simulink model "Android_interface_2Aero"  (R2018b)
settings: Solver=FixedStepDiscrete  StartTime=0.0  StopTime=inf  FixedStep=0.002  RelTol=1e-3
libraries: androiduilib x8, androidcommunicationlib x8
settings Model: SimulationMode=external  ExtModeTrigDuration=10000  Creator=gjaniak  LastModifiedBy=gjaniak
settings SolverCC: PositivePriorityOrder=on
settings OptimizationCC: PassReuseOutputArgsThreshold=0  MaxStackSize=64
settings DebuggingCC: ParameterTunabilityLossMsg=error  LibraryContextMissingDiagnostic=none
settings HardwareCC: ProdBitPerPointer=32  ProdBitPerSizeT=32  ProdBitPerPtrDiffT=32  ProdLargestAtomicInteger=Long  ProdLargestAtomicFloat=Double  ProdWordSize=32  ProdHWDeviceType=ARM Compatible->ARM Cortex  UseEmbeddedCoderFeatures=off
settings SFSimCC: SimUseLocalCustomCode=off
settings RTWCC: SystemTargetFile=ert.tlc  HardwareBoard=Android Device  TLCOptions="-aInlineSetEventsForThisBaseRateFcn=TLC_FALSE -aSuppressMultiTaskScheduler=TLC_FALSE  -aRateBasedStepFcn=0"  TemplateMakefile=ert_default_tmf  GenerateReport=on  RTWUseLocalCustomCode=off  Toolchain=Android SDK/NDK Tools  LaunchReport=on
settings CodeAppCC: ForceParamTrailComments=on  OperatorAnnotations=on  StateflowObjectComments=on  MATLABSourceComments=on
settings ERTTargetCC: MultiwordLength=2048  ERTCustomFileBanners=off  SupportContinuousTime=on  SupportNonInlinedSFcns=on  RemoveResetFunc=off  ModelStepFunctionPrototypeControlCompliant=off

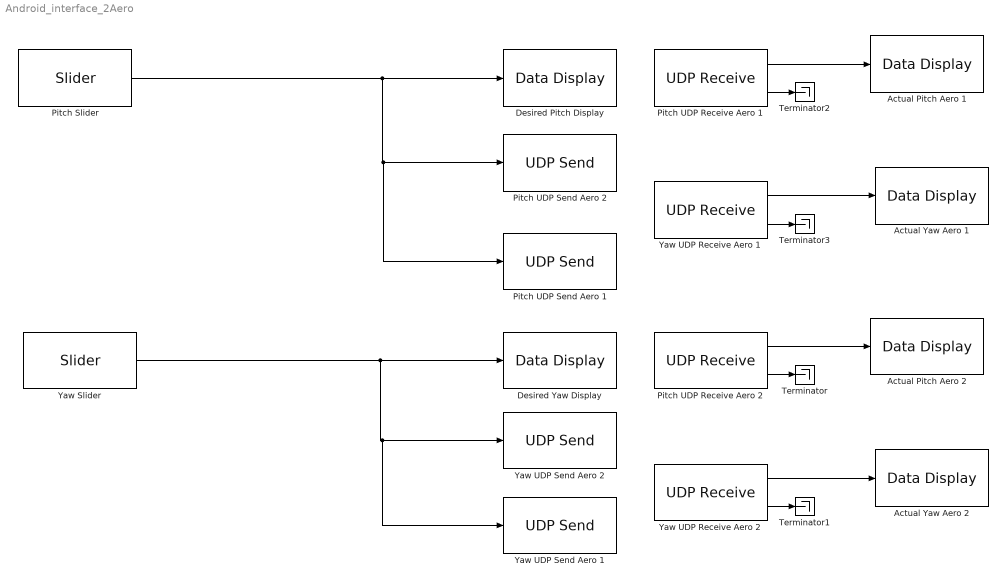
== system Android_interface_2Aero ==
  Actual Pitch Aero 1 : androiduilib/Data Display  DataDisplayId=Android_interface_2Aero/Actual_Pitch_Aero_1  Format=Float  Precision=6  SimulateUsing=Code generation  blockPlatform=Android
      settings: SourceProductName=Simulink Support Package for Android Devices  SourceProductBaseCode=ANDROID
  Actual Pitch Aero 2 : androiduilib/Data Display  DataDisplayId=Android_interface_2Aero/Actual_Pitch_Aero_2  Format=Float  Precision=6  SimulateUsing=Code generation  blockPlatform=Android
      settings: SourceProductName=Simulink Support Package for Android Devices  SourceProductBaseCode=ANDROID
  Actual Yaw Aero 1 : androiduilib/Data Display  DataDisplayId=Android_interface_2Aero/Actual_Yaw_Aero_1  Format=Float  Precision=6  SimulateUsing=Code generation  blockPlatform=Android
      settings: SourceProductName=Simulink Support Package for Android Devices  SourceProductBaseCode=ANDROID
  Actual Yaw Aero 2 : androiduilib/Data Display  DataDisplayId=Android_interface_2Aero/Actual_Yaw_Aero_2  Format=Float  Precision=6  SimulateUsing=Code generation  blockPlatform=Android
      settings: SourceProductName=Simulink Support Package for Android Devices  SourceProductBaseCode=ANDROID
  Desired Pitch Display : androiduilib/Data Display  DataDisplayId=Android_interface_2Aero/Desired_Pitch_Display  Format=Float  Precision=6  SimulateUsing=Code generation  blockPlatform=Android
      settings: SourceProductName=Simulink Support Package for Android Devices  SourceProductBaseCode=ANDROID
  Desired Yaw Display : androiduilib/Data Display  DataDisplayId=Android_interface_2Aero/Desired_Yaw_Display  Format=Float  Precision=6  SimulateUsing=Code generation  blockPlatform=Android
      settings: SourceProductName=Simulink Support Package for Android Devices  SourceProductBaseCode=ANDROID
  Pitch Slider : androiduilib/Slider  Min=-60  Value=0  Max=60  Resolution=1  SliderId=Android_interface_2Aero/Pitch_Slider  SampleTime=0.1  BlockPlatform=Android
      settings: SourceProductName=Simulink Support Package for Android Devices  SourceProductBaseCode=ANDROID
  Pitch UDP Receive Aero 1 : androidcommunicationlib/UDP Receive  localURL='0.0.0.0'  localPort=26004  remoteURL='0.0.0.0'  remotePort=-1  recvBufferSize=8192  signalDatatype=double  dims=1  isVarSize=off  showBlockingTime=off  blockingTime=0  sampletime=0.01  blockPlatform=Android
      settings: SourceProductName=Simulink Support Package for Android Devices  SourceProductBaseCode=ANDROID
  Pitch UDP Receive Aero 2 : androidcommunicationlib/UDP Receive  localURL='0.0.0.0'  localPort=26002  remoteURL='0.0.0.0'  remotePort=-1  recvBufferSize=8192  signalDatatype=double  dims=1  isVarSize=off  showBlockingTime=off  blockingTime=0  sampletime=0.01  blockPlatform=Android
      settings: SourceProductName=Simulink Support Package for Android Devices  SourceProductBaseCode=ANDROID
  Pitch UDP Send Aero 1 : androidcommunicationlib/UDP Send  remoteURL='192.168.1.79'  remotePort=26006  localURL='0.0.0.0'  localPortSource=Automatically determine  localPort=-1  sampletime=-1  blockPlatform=Android  separateLengthPort=0
      settings: SourceProductName=Simulink Support Package for Android Devices  SourceProductBaseCode=ANDROID
  Pitch UDP Send Aero 2 : androidcommunicationlib/UDP Send  remoteURL='192.168.1.20'  remotePort=26000  localURL='0.0.0.0'  localPortSource=Automatically determine  localPort=-1  sampletime=-1  blockPlatform=Android  separateLengthPort=0
      settings: SourceProductName=Simulink Support Package for Android Devices  SourceProductBaseCode=ANDROID
  Terminator{,1..3} (4 alike) : Terminator
  Yaw Slider : androiduilib/Slider  Min=-180  Value=0  Max=180  Resolution=1  SliderId=Android_interface_2Aero/Yaw_Slider  SampleTime=0.1  BlockPlatform=Android
      settings: SourceProductName=Simulink Support Package for Android Devices  SourceProductBaseCode=ANDROID
  Yaw UDP Receive Aero 1 : androidcommunicationlib/UDP Receive  localURL='0.0.0.0'  localPort=26005  remoteURL='0.0.0.0'  remotePort=-1  recvBufferSize=8192  signalDatatype=double  dims=1  isVarSize=off  showBlockingTime=off  blockingTime=0  sampletime=0.01  blockPlatform=Android
      settings: SourceProductName=Simulink Support Package for Android Devices  SourceProductBaseCode=ANDROID
  Yaw UDP Receive Aero 2 : androidcommunicationlib/UDP Receive  localURL='0.0.0.0'  localPort=26003  remoteURL='0.0.0.0'  remotePort=-1  recvBufferSize=8192  signalDatatype=double  dims=1  isVarSize=off  showBlockingTime=off  blockingTime=0  sampletime=0.01  blockPlatform=Android
      settings: SourceProductName=Simulink Support Package for Android Devices  SourceProductBaseCode=ANDROID
  Yaw UDP Send Aero 1 : androidcommunicationlib/UDP Send  remoteURL='192.168.1.79'  remotePort=26007  localURL='0.0.0.0'  localPortSource=Automatically determine  localPort=-1  sampletime=-1  blockPlatform=Android  separateLengthPort=0
      settings: SourceProductName=Simulink Support Package for Android Devices  SourceProductBaseCode=ANDROID
  Yaw UDP Send Aero 2 : androidcommunicationlib/UDP Send  remoteURL='192.168.1.20'  remotePort=26001  localURL='0.0.0.0'  localPortSource=Automatically determine  localPort=-1  sampletime=-1  blockPlatform=Android  separateLengthPort=0
      settings: SourceProductName=Simulink Support Package for Android Devices  SourceProductBaseCode=ANDROID
  wires:
  Yaw UDP Receive Aero 2/1 -> Actual Yaw Aero 2/1
  Pitch UDP Receive Aero 2/1 -> Actual Pitch Aero 2/1
  Yaw Slider/1 -> Yaw UDP Send Aero 1/1, Yaw UDP Send Aero 2/1, Desired Yaw Display/1
  Pitch Slider/1 -> Pitch UDP Send Aero 1/1, Pitch UDP Send Aero 2/1, Desired Pitch Display/1
  Pitch UDP Receive Aero 2/2 -> Terminator/1
  Yaw UDP Receive Aero 2/2 -> Terminator1/1
  Pitch UDP Receive Aero 1/1 -> Actual Pitch Aero 1/1
  Yaw UDP Receive Aero 1/2 -> Terminator3/1
  Pitch UDP Receive Aero 1/2 -> Terminator2/1
  Yaw UDP Receive Aero 1/1 -> Actual Yaw Aero 1/1
